simulink model "XX_2016a"  (R2016a)
settings: Solver=VariableStepAuto  SolverMode=SingleTasking  StartTime=0.0  StopTime=10.0  RelTol=1e-3
values from neighbouring files (symbols this model uses):
  g = 9.81    [Uebung1.m]
  m = 10    [Uebung1.m]    (also in Uebung11.m)
undefined symbols (not defined in the file or in its folder): A, c_w, dkv_lookup, i_D, i_G, k_r, M_mot_m_lookup, m_rot, q, r, roh, w_all_m_lookup
settings Model: Creator=Jason  LastModifiedBy=Jason
settings DebuggingCC: SFUnexpectedBacktrackingDiag=error  SFNoUnconditionalDefaultTransitionDiag=error
settings GRTTargetCC: TargetLangStandard=C99 (ISO)  GeneratePreprocessorConditionals=Use local settings
settings ConfigComp: CovMetricSettings=dwe  CovHtmlReporting=off  CovSaveCumulativeToWorkspaceVar=off  CovSaveSingleToWorkspaceVar=off  CovExternalEMLEnable=on

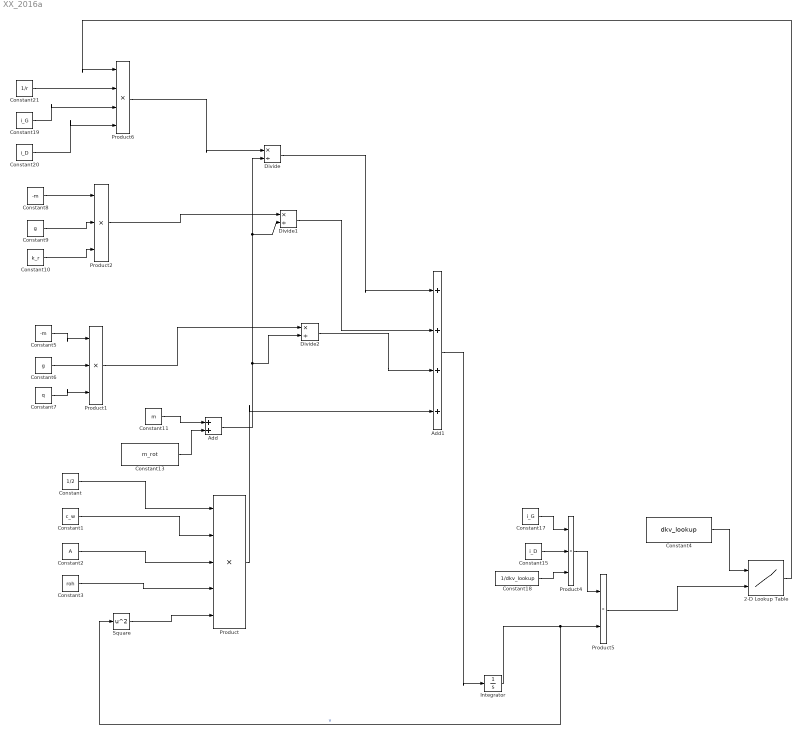
== system XX_2016a ==
  2-D Lookup Table : Lookup_n-D  BreakpointsForDimension1=dkv_lookup  BreakpointsForDimension2=w_all_m_lookup  Table=M_mot_m_lookup  InternalRulePriority=Speed  RndMeth=Simplest  InputSameDT=on
  Add : Sum
  Add1 : Sum  Inputs=++++
  Constant : Constant  Value=1/2
  Constant1 : Constant  Value=c_w
  Constant10 : Constant  Value=k_r
  Constant11 : Constant  Value=m
  Constant13 : Constant  Value=m_rot
  Constant15 : Constant  Value=i_D
  Constant17 : Constant  Value=i_G
  Constant18 : Constant  Value=1/dkv_lookup
  Constant19 : Constant  Value=i_G
  Constant2 : Constant  Value=A
  Constant20 : Constant  Value=i_D
  Constant21 : Constant  Value=1/r
  Constant3 : Constant  Value=roh
  Constant4 : Constant  Value=dkv_lookup
  Constant5 : Constant  Value=-m
  Constant6 : Constant  Value=g
  Constant7 : Constant  Value=q
  Constant8 : Constant  Value=-m
  Constant9 : Constant  Value=g
  Divide : Product  Inputs=*/
  Divide1 : Product  Inputs=*/
  Divide2 : Product  Inputs=*/
  Integrator : Integrator
  Product : Product  Inputs=5
  Product1 : Product  Inputs=3
  Product2 : Product  Inputs=3
  Product4 : Product  Inputs=3
  Product5 : Product
  Product6 : Product  Inputs=4
  Square : Math  Operator=square  SaturateOnIntegerOverflow=on
  wires:
  Constant/1 -> Product/1
  Constant3/1 -> Product/4
  Square/1 -> Product/5
  Constant1/1 -> Product/2
  Constant2/1 -> Product/3
  Constant5/1 -> Product1/1
  Constant6/1 -> Product1/2
  Constant7/1 -> Product1/3
  Constant8/1 -> Product2/1
  Constant9/1 -> Product2/2
  Constant10/1 -> Product2/3
  Constant11/1 -> Add/1
  Constant13/1 -> Add/2
  Integrator/1 -> Square/1, Product5/2  "v"
  Constant4/1 -> 2-D Lookup Table/1
  Constant17/1 -> Product4/1
  Constant15/1 -> Product4/2
  Constant18/1 -> Product4/3
  Product4/1 -> Product5/1
  Product5/1 -> 2-D Lookup Table/2
  Constant21/1 -> Product6/2
  Constant19/1 -> Product6/3
  Constant20/1 -> Product6/4
  Product6/1 -> Divide/1
  Add/1 -> Divide2/2, Divide/2, Divide1/2
  Product2/1 -> Divide1/1
  Product1/1 -> Divide2/1
  Divide/1 -> Add1/1
  Divide1/1 -> Add1/2
  Divide2/1 -> Add1/3
  Product/1 -> Add1/4
  Add1/1 -> Integrator/1
  2-D Lookup Table/1 -> Product6/1
